simulink model "methode_des_moyennes"  (R2023b)
settings: Solver=VariableStepAuto  StartTime=0.0  StopTime=50  FixedStep=0.01  RelTol=1e-3
libraries: spsMeanLib x2
settings Model: Creator=matth  LastModifiedBy=matth

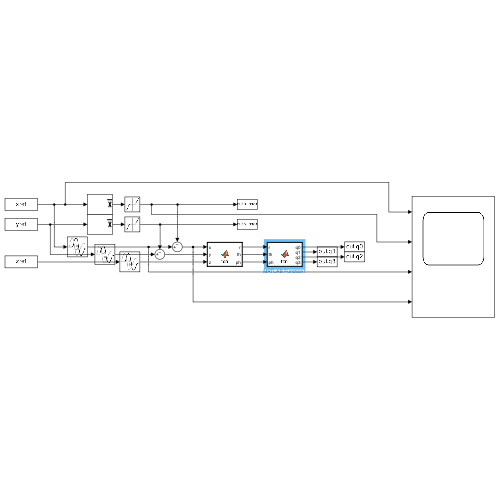
[thumbnail: Simulink's stored preview of the top-level diagram]
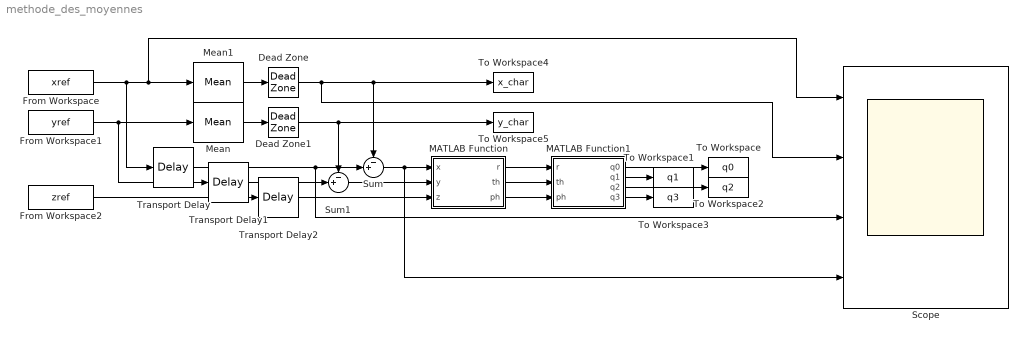
== system methode_des_moyennes ==
  Dead Zone : DeadZone  LowerValue=-0.01  UpperValue=0.01
  Dead Zone1 : DeadZone  LowerValue=-0.01  UpperValue=0.01
  From Workspace : FromWorkspace  VariableName=xref
  From Workspace1 : FromWorkspace  VariableName=yref
  From Workspace2 : FromWorkspace  VariableName=zref
  MATLAB Function : MATLAB Function  TreatAsAtomicUnit=on
  MATLAB Function1 : MATLAB Function  TreatAsAtomicUnit=on
  Mean : spsMeanLib/Mean  Freq=60  Vinit=0  Ts=0
  Mean1 : spsMeanLib/Mean  Freq=2/pi  Vinit=0  Ts=0
  Scope : Scope  NumInputPorts=4
  Sum : Sum  Inputs=-+|
  Sum1 : Sum  Inputs=-+|
  To Workspace : ToWorkspace  VariableName=q0  SaveFormat=Structure With Time  SampleTime=-1
  To Workspace1 : ToWorkspace  VariableName=q1  SaveFormat=Structure With Time  SampleTime=-1
  To Workspace2 : ToWorkspace  VariableName=q2  SaveFormat=Structure With Time  SampleTime=-1
  To Workspace3 : ToWorkspace  VariableName=q3  SaveFormat=Structure With Time  SampleTime=-1
  To Workspace4 : ToWorkspace  VariableName=x_char  SaveFormat=Structure With Time  SampleTime=-1
  To Workspace5 : ToWorkspace  VariableName=y_char  SaveFormat=Structure With Time  SampleTime=-1
  Transport Delay : TransportDelay  DelayTime=pi/2
  Transport Delay1 : TransportDelay  DelayTime=pi/2
  Transport Delay2 : TransportDelay  DelayTime=pi/2
  wires:
  Mean/1 -> Dead Zone1/1
  Mean1/1 -> Dead Zone/1
  MATLAB Function/1(r) -> MATLAB Function1/1(r)
  MATLAB Function/2(th) -> MATLAB Function1/2(th)
  MATLAB Function/3(ph) -> MATLAB Function1/3(ph)
  Dead Zone/1 -> Scope/2, Sum/1, To Workspace4/1
  Dead Zone1/1 -> Sum1/1, To Workspace5/1
  Sum/1 -> Scope/4, MATLAB Function/1(x)
  Sum1/1 -> MATLAB Function/2(y)
  From Workspace/1 -> Transport Delay/1, Scope/1, Mean1/1
  From Workspace1/1 -> Mean/1, Transport Delay1/1
  From Workspace2/1 -> Transport Delay2/1
  MATLAB Function1/1(q0) -> To Workspace/1
  MATLAB Function1/2(q1) -> To Workspace1/1
  MATLAB Function1/3(q2) -> To Workspace2/1
  MATLAB Function1/4(q3) -> To Workspace3/1
  Transport Delay/1 -> Scope/3, Sum/2
  Transport Delay1/1 -> Sum1/2
  Transport Delay2/1 -> MATLAB Function/3(z)

== matlab function methode_des_moyennes/MATLAB Function1 ==
  data: r input; q0 output; th input; ph input; q1 output; q2 output; q3 output
function [q0,q1,q2,q3] = fcn(r, th, ph)

    [q0,q1,q2,q3] = trouve_pos_ang_sph(r,th,ph);

== matlab function methode_des_moyennes/MATLAB Function ==
  data: x input; r output; y input; z input; th output; ph output
function [r, th, ph] = fcn(x, y, z)

[r, th, ph] = changement_base(x, y, z);
